simulink model "momentumBasedFlying"  (Simulink 10.3)
settings: Solver=FixedStepAuto  StartTime=0.0  StopTime=Config.simulationTime  FixedStep=Config.tStep  RelTol=1e-3
InitFcn:
  | cd(fileparts(which(bdroot)));
  | initMomentumBasedFlying;
StopFcn:
  | cd(fileparts(which(bdroot)));
  | stopMomentumBasedFlying;
undefined symbols (not defined in the file): biasVectorConstraint_feet, Config, confVisualizer, ConstraintMatrix_feet, DiscIntNeverNeededParam, jets_config
libraries: WBToolboxLibrary x75
(part 4 of 4)

== matlab function FLYING CONTROLLER (CORE) V2.5/Flight Controller RAL-HUMANOIDS V3.1/Momentum Control for Flying/QP Solver and Integrate Contact Forces Derivative/Integrate the Contact Forces Derivative/Select Integrator Initial Condition ==
  data: feetContactIsActive input double; contactForces input double; contactForces_0 output double
function contactForces_0 = selectInitContactForcesFCN(feetContactIsActive, contactForces)

    contactForces_0 = iRonCubLib.selectInitContactForces(feetContactIsActive, contactForces);
end

== matlab function JoyStick Commands/JoyStick-flightGUI Commands/Replace Joystick with Native GUI ==
  data: gui_input input double; joyButtons output double; joyAxes output double
function [joyButtons,joyAxes] = fromGuiToJoystickFCN(gui_input)

    [joyButtons,joyAxes] = iRonCubLib.fromGuiToJoystick(gui_input);
end

== matlab function FLYING CONTROLLER (CORE) V2.5/Flight Controller RAL-HUMANOIDS V3.1/Momentum Control for Flying/QP Solver and Integrate Contact Forces Derivative/Integrate the Contact Forces Derivative/deadZone/Deadzone Function ==
  data: u input double; y output double; thr input double
function y = deadZoneFCN(u, thr)

    y = wbc.deadZone(u, thr);
end

== matlab function FLYING CONTROLLER (CORE) V2.5/Flight Controller RAL-HUMANOIDS V3.1/Momentum Control for Flying/QP Solver and Integrate Contact Forces Derivative/QP momentumControl/Process QP Inputs Momentum Control ==
  data: HessianMatrixQP input double; H_balancing output double; gVectorQP input double; lowerBoundQP input double; upperBoundQP input double; g_balancing output double; ub_balancing output double; lb_balancing output double; H_flight output double; g_flight output double; ub_flight output double; lb_flight output double
function [H_balancing,g_balancing,ub_balancing,lb_balancing, ...
          H_flight,g_flight,ub_flight,lb_flight] = processQPinputMomentumControlFCN(HessianMatrixQP,gVectorQP,lowerBoundQP,upperBoundQP) 
      
    [H_balancing,g_balancing,ub_balancing,lb_balancing, ...
        H_flight,g_flight,ub_flight,lb_flight] = iRonCubLib.processQPinputMomentumControl(HessianMatrixQP,gVectorQP,lowerBoundQP,upperBoundQP);
end

== matlab function FLYING CONTROLLER (CORE) V2.5/Flight Controller RAL-HUMANOIDS V3.1/Momentum Control for Flying/Feedback linearization/MATLAB Function ==
  data: jets input double; jets_dot input double; jets_dot_des input double; throttle output double size=[4,1]; Config parameter double; error output double; integral_err input double
function [throttle, error]  = fl_jet_control(jets, jets_dot, jets_dot_des, Config, integral_err)

[throttle, error]  = fl_jet_control(jets, jets_dot, jets_dot_des, Config, integral_err);
end

== matlab function FLYING CONTROLLER (CORE) V2.5/Flight Controller RAL-HUMANOIDS V3.1/Momentum Control for Flying/extendedKalmanFilter4jets/EKF_jet1/EKF  ==
  data: x input double; input input double; measurement input double; xDot output double; P input double; Config parameter double; Pdot output double
function [xDot, Pdot] = extendedKalmanFilterFNC(x, input, measurement, P, Config)

[xDot, Pdot] = extKalmanFilter(x, input, Config.jetC_P100, P, measurement, Config);

== matlab function FLYING CONTROLLER (CORE) V2.5/Flight Controller RAL-HUMANOIDS V3.1/Momentum Control for Flying/extendedKalmanFilter4jets/EKF_jet1/splitVector ==
  data: x input double; x1 output double; x2 output double
function [x1, x2] = fcn(x)
x1 = x(1);
x2 = x(2);

== matlab function FLYING CONTROLLER (CORE) V2.5/Flight Controller RAL-HUMANOIDS V3.1/Momentum Control for Flying/extendedKalmanFilter4jets/EKF_jet2/EKF  ==
  data: x input double; input input double; measurement input double; xDot output double; P input double; Config parameter double; Pdot output double
function [xDot, Pdot] = extendedKalmanFilterFNC(x, input, measurement, P, Config)

[xDot, Pdot] = extKalmanFilter(x, input, Config.jetC_P100, P, measurement, Config);

== matlab function FLYING CONTROLLER (CORE) V2.5/Flight Controller RAL-HUMANOIDS V3.1/Momentum Control for Flying/extendedKalmanFilter4jets/EKF_jet2/splitVector ==
  data: x input double; x1 output double; x2 output double
function [x1, x2] = fcn(x)
x1 = x(1);
x2 = x(2);

== matlab function FLYING CONTROLLER (CORE) V2.5/Flight Controller RAL-HUMANOIDS V3.1/Momentum Control for Flying/extendedKalmanFilter4jets/EKF_jet3/EKF  ==
  data: x input double; input input double; measurement input double; xDot output double; P input double; Config parameter double; Pdot output double
function [xDot, Pdot] = extendedKalmanFilterFNC(x, input, measurement, P, Config)

[xDot, Pdot] = extKalmanFilter(x, input, Config.jetC_P220, P, measurement, Config);

== matlab function FLYING CONTROLLER (CORE) V2.5/Flight Controller RAL-HUMANOIDS V3.1/Momentum Control for Flying/extendedKalmanFilter4jets/EKF_jet3/splitVector ==
  data: x input double; x1 output double; x2 output double
function [x1, x2] = fcn(x)
x1 = x(1);
x2 = x(2);

== matlab function FLYING CONTROLLER (CORE) V2.5/Flight Controller RAL-HUMANOIDS V3.1/Momentum Control for Flying/extendedKalmanFilter4jets/EKF_jet4/EKF  ==
  data: x input double; input input double; measurement input double; xDot output double; P input double; Config parameter double; Pdot output double
function [xDot, Pdot] = extendedKalmanFilterFNC(x, input, measurement, P, Config)

[xDot, Pdot] = extKalmanFilter(x, input, Config.jetC_P220, P, measurement, Config);

== matlab function FLYING CONTROLLER (CORE) V2.5/Flight Controller RAL-HUMANOIDS V3.1/Momentum Control for Flying/extendedKalmanFilter4jets/EKF_jet4/splitVector ==
  data: x input double; x1 output double; x2 output double
function [x1, x2] = fcn(x)
x1 = x(1);
x2 = x(2);
